simulink model "Sim_Control_Dezvoltare"  (R2022b)
settings: Solver=VariableStepAuto  StartTime=0.0  StopTime=400  RelTol=1e-3
values from neighbouring files (symbols this model uses):
  g = 9.80665    [Date_initializare_SIM.m]
  h = 0.30    (= 0.3)    [Date_initializare_SIM.m]
undefined symbols (not defined in the file or in its folder): X, Y, Z
libraries: sm_lib x175, nesl_utility x70, slpidlib x2
(part 5 of 5)

== matlab function Sim_Control_Dezvoltare/MATLAB Function7 ==
  data: pstar input size=[3,1]; q_bl output size=[1,3]; Tx input; Ty input; Tz input; Rx input; Ry input; Rz input
function q_bl = ikine_rl_f(pstar, Tx, Ty, Tz, Rx, Ry, Rz)
  
    R_DH = rotz(0)*roty(90)*rotx(0);
    T_DH = [0; 0; 0];
    O_DH = [R_DH, T_DH; [0 0 0 1] ];
    
    R_fr = rotz(0)*rotx(0);
    T_fr = [0; 0.047; -0.1805];
    O_fr = [R_fr, T_fr; [0 0 0 1] ];
    
    R_c_corp = rotz(Rx)*roty(Ry)*rotx(Rz);
    T_c_corp = [-Tz; Ty; Tx];
    O_c_corp = [R_c_corp, T_c_corp; [0 0 0 1] ];
        
    B =  O_DH * O_c_corp * O_fr;
    
    pzero = [B(1,4), B(2,4), B(3,4)];
    
    x0_ = pzero(1);
    y0_ = pzero(2);
    z0_ = pzero(3);
    
    x_ = pstar(1);
    y_ = pstar(2);
    z_ = pstar(3);

    Rot = [rotz(Rz)*roty(-Ry)*rotx(-Rx), [0; 0; 0]; [0 0 0 1]];
    Point = [1 0 0 x_-x0_; 0 1 0 y_-y0_; 0 0 1 z_-z0_; 0 0 0 1];
    Origin = [1 0 0 x0_; 0 1 0 y0_; 0 0 1 z0_; 0 0 0 1];
    
    pstar = Origin + Rot*Point;

    x_ = pstar(1,4);
    y_ = pstar(2,4);
    z_ = pstar(3,4);


%     d = sqrt((x_ - x0_)*(x_ - x0_) + (y_ - y0_)*(y_ - y0_) + (z_ - z0_)*(z_ - z0_));
% 
%     th = acos((z_ - z0_)/d) 
%     fis = acos((x_ - x0_)/(d*sin(th)))% + Rz*2*pi/360
% 
%     star = [x0_; y0_; z0_] + rotx(Rx)*roty(-Ry)*rotz(Rz)*(d.*[cos(fis)*sin(th); sin(fis)*sin(th); cos(th)]) 
%     
%     x_ = star(1)
%     y_ = star(2)
%     z_ = star(3)

    
    off = 0.0838;
    L = 0.2;

    m = sqrt((z_ - z0_)*(z_ - z0_));
    n = sqrt( (y_ - y0_)*(y_ - y0_));
    p = sqrt( (y0_ - y_)*(y0_ - y_) + (z0_ - z_)*(z0_ - z_));
    alp0 = atan(n/m);
    alp1 = asin(off/p);
    q1_ = (alp0 - alp1) ;

    x = sqrt((x_ - x0_)*(x_ - x0_));
    r = sqrt(p*p - off*off);
    a = sqrt(r*r + x*x);

    fi = asin((x_ - x0_)/a);

    alpha = acos((a*a + L*L - L*L)/(2*a*L));
    q2_ =  alpha - fi ;
    q3_ = -pi + acos((L*L + L*L - a*a)/(2*L*L)) ;

    q_bl = [q1_, q2_, q3_];

end

== matlab function Sim_Control_Dezvoltare/MATLAB Function18 ==
  data: Fr input; Fl input; centroid output; Rr input; Rl input; pfr input; prl input; prr input; pfl input; rx input; ry input; rz input; rot output
function [centroid, rot]= centroid(Fr, Fl, Rr, Rl, pfr, prl, prr, pfl, rx, ry, rz)

Rot = rotx(rx)*roty(ry)*rotz(rz);
centroid  = (1/(prl + pfl + pfr + prr).*(prl.*Rl + prr.*Rr + pfr.*Fr + pfl.*Fl));
rot = [rx, ry, rz];




end

== matlab function Sim_Control_Dezvoltare/MATLAB Function22 ==
  data: X1 output; A input; B input; t input; d input
function X1 = Traj(A, B, t, d)
  
% t = -1:0.01:1;
% A = [1, 1, 8]';
% B = [1, 10, 8]';


C = 1/2*(A + B);
D = C + [0, 0, d]';

X1 = C + (C - A)*t + (D-C)*(1-t^2);



end

== matlab function Sim_Control_Dezvoltare/MATLAB Function23 ==
  data: X output; A input; B input; t input; d input
function X = Traj(A, B, t, d)
  
% t = -1:0.01:1;
% A = [1, 1, 8]';
% B = [1, 10, 8]';


C = 1/2*(A + B);
D = C + [0, 0, d]';

X = C + (C - A)*t + (D-C)*(1-t^2);



end

== matlab function Sim_Control_Dezvoltare/MATLAB Function24 ==
  data: X output; A input; B input; t input; d input
function X = Traj(A, B, t, d)
  
% t = -1:0.01:1;
% A = [1, 1, 8]';
% B = [1, 10, 8]';


C = 1/2*(A + B);
D = C + [0, 0, d]';

X = C + (C - A)*t + (D-C)*(1-t^2);



end

== matlab function Sim_Control_Dezvoltare/MATLAB Function25 ==
  data: step input; traj output size=[1,2]
function traj = fcn(step)
    
    if step == 0
        step = 1;
    end
    %x = 0:3:1000;
    x = linspace(0,300,100);
    y = 0:0.3:60;
    
    traj = [x(step),0];


end

== matlab function Sim_Control_Dezvoltare/MATLAB Function26 ==
  data: X input; Tx output; Ty output; Tz output; Y input; Z input; R input; Rx output; Ry output; Rz output
function [Tx, Ty, Tz, Rx, Ry, Rz]= Corp(X, Y, Z, R)

Tx = X;
Ty = Y;
Tz = Z;

Rx = R(1,1);
Ry = R(1,2);
Rz = R(1,3);

end

== matlab function Sim_Control_Dezvoltare/MATLAB Function28 ==
  data: X output; A input; B input; t input; d input
function X = Traj(A, B, t, d)
  
% t = -1:0.01:1;
% A = [1, 1, 8]';
% B = [1, 10, 8]';

C = 1/2*(A + B);
D = C + [0, 0, d]';

X = C + (C - A)*t + (D-C)*(1-t^2);



end

== stateflow chart Sim_Control_Dezvoltare/Step Planning Logic3 ==
  settings: updateMethod=DISCRETE  sampleTime=0.1
  state control [function]
    (default) -> (junction 43) : {
        | footRH_prev =  footRH;
        | footLH_prev =  footLH;
        | footRB_prev =  footRB;
        | footLB_prev =  footLB;
        | RH = offRH + [xrefRH;yrefRH;zrefRH];
        |
        | Rot = rotx(rx_out)*roty(ry_out)*rotz(rz_out);
        |
        | footRH = (Rot*RH)
        | }
  state control1 [function]
    (default) -> (junction 139) : {
        | footRH_prev =  footRH;
        | footLH_prev =  footLH;
        | footRB_prev =  footRB;
        | footLB_prev =  footLB;
        |
        | LB = offLB + [xrefLB;yrefLB;zrefLB];
        | Rot = rotx(rx_out)*roty(ry_out)*rotz(rz_out);
        |
        | footLB = (Rot*LB);
        | }
  state control2 [function]
    (default) -> (junction 245) : {
        |
        | footRH_prev =  footRH;
        | footLH_prev =  footLH;
        | footRB_prev =  footRB;
        | footLB_prev =  footLB;
        |
        | LH = offLH + [xrefLH;yrefLH;zrefLH];
        |
        | Rot = rotx(rx_out)*roty(ry_out)*rotz(rz_out);
        | footLH = (Rot*LH);
        |
        | }
  state control3 [function]
    (default) -> (junction 249) : {
        |
        | footRH_prev =  footRH;
        | footLH_prev =  footLH;
        | footRB_prev =  footRB;
        | footLB_prev =  footLB;
        |
        | RB = offRB + [xrefRB;yrefRB;zrefRB];
        | Rot = rotx(rx_out)*roty(ry_out)*rotz(rz_out);
        |
        | footRB = (Rot*RB);
        |
        | }
  state test8
  state Initial
    t = -1;
    timp_traj = t;
    dRH = 0;
    dLB = 0;
    dRB = 0;
    dLH = 0;
    prr = 1;
    prl = 1;
    pfr = 1;
    pfl = 1;
    rx_out = 0.001;
    ry_out = 0.001;
    rz_out = 0.001;
    control;
    control1;
    control2;
    control3;
  state test4
    step = step+1;
  state RightFrontFoot
    xrefRH = stepFwd;
    yrefRH = max(0,stepLat);
    dRH = 0;
    dLB = 0;
    dRB = 0;
    dLH = 0;
    prr = 1;
    prl = 1;
    pfr = 0;
    pfl = 1;
    t = -1;
    rx_out = rx;
    ry_out = ry;
    rz_out = rz;
    timp_traj = t;
    control
  state LeftBackFoot
    xrefLB = stepFwd;
    yrefLB = max(0,stepLat);
    dRH = 0;
    dLB = 0;
    dRB = 0;
    dLH = 0;
    prr = 1;
    prl = 0;
    pfr = 1;
    pfl = 1;
    t = -1;
    timp_traj = t;
    control1
  state timp
    if t<1
    dRH = hs;
    dLB = 0;
    dRB = 0;
    dLH = 0;
    t = t + increment;
    timp_traj = t;
    end
    %if t>=1
    %  if t~=1
    %      t = 1;
    %    timp_traj = t;
    % else
    %   timp_traj = timp_traj + inc
    %end
    %end
  state test
    after(1,sec)
  state test7
    step = step+1;
  state timp1
    if t<1
    dRH = 0;
    dLB = 0;
    dRB = hs;
    dLH = 0;
    t = t + increment;
    timp_traj = t;
    end
  state test1
    after(1,sec)
  state timp2
    if t<1
    dRH = 0;
    dLB = hs;
    dRB = 0;
    dLH = 0;
    t = t + increment;
    timp_traj = t;
    end
  state test6
    step = step+1;
  state test5
    after(1,sec)
  state LeftFrontFoot
    xrefLH = stepFwd;
    yrefLH = max(0,stepLat);
    dRH = 0;
    dLB = 0;
    dRB = 0;
    dLH = 0;
    prr = 1;
    prl = 1;
    pfr = 1;
    pfl = 0;
    t = -1;
    rx_out = rx;
    ry_out = ry;
    rz_out = rz;
    timp_traj = t;
    control2
  state timp3
    if t<1
    dRH = 0;
    dLB = 0;
    dRB = 0;
    dLH = hs;
    t = t + increment;
    timp_traj = t;
    end
  state RightBackFoot
    xrefRB = stepFwd;
    yrefRB= max(0,stepLat);
    dRH = 0;
    dLB = 0;
    dRB = 0;
    dLH = 0;
    prr = 0;
    prl = 1;
    pfr = 1;
    pfl = 1;
    t = -1;
    timp_traj = t;
    control3
  state test2
    after(1,sec)
  (default) -> test8 : % Initialize values
      | {
      | offRH = [0.1805; -0.047-0.0838; -0.3];
      | offLH = [0.1805; 0.047+0.0838; -0.3];
      | offRB = [-0.1805; -0.047-0.0838; -0.3];
      | offLB = [-0.1805; 0.047+0.0838; -0.3];
      | footRH = (offRH);
      | footLH = (offLH);
      | footRB = (offRB);
      | footLB = (offLB);
      | footRH_prev = (offRH);
      | footLH_prev = (offLH);
      | footRB_prev = (offRB);
      | footLB_prev = (offLB);
      |
      | hs = 0.1;
      |
      | tol = 0.01;
      | inc = 0.001;
      | increment = 0.5;
      | t = -1;
      | timp_traj = t;
      | dRH = 0;
      | dLB = 0;
      | dRB = 0;
      | dLH = 0;
      | prr = 1;
      | prl = 1;
      | pfr = 1;
      | pfl = 1;
      | xrefLH = 0; yrefLH = 0; zrefLH = 0;
      | xrefRH = 0; yrefRH = 0; zrefRH = 0;
      | xrefLB = 0; yrefLB = 0; zrefLB = 0;
      | xrefRB = 0; yrefRB = 0; zrefRB = 0;
      | step = 1;
      | rx_out = 0.001;
      | ry_out = 0.001;
      | rz_out = 0.001;
      |
      | control;
      | control1;
      | control2;
      | control3;
      |
      | }
  test8 -> Initial
  Initial -> test4
  test4 -> RightFrontFoot : [err_cg<tol ]
  timp -> timp [order 1] : [ presFR==0]
  test -> timp : [err_cg<tol]
  RightFrontFoot -> test
  timp -> LeftBackFoot [order 2] : [ presFR>0 && t>=1]
  LeftBackFoot -> test1
  test7 -> RightFrontFoot
  timp2 -> timp2 [order 1] : [presRL==0]
  timp1 -> test7 [order 1] : [presRR>0 && t>=1]
  test1 -> timp2 : [err_cg<tol ]
  timp2 -> test6 [order 2] : [ presRL>0 && t>=1]
  test5 -> timp1 : [err_cg<tol ]
  timp1 -> timp1 [order 2] : [presRR==0]
  test6 -> LeftFrontFoot
  RightBackFoot -> test5
  timp3 -> timp3 [order 1] : [presFL==0]
  timp3 -> RightBackFoot [order 2] : [presFL>0 && t>=1]
  test2 -> timp3 : [err_cg<tol]
  LeftFrontFoot -> test2
  data: footRH output size=[3,1]; footLH output size=[3,1]; stepFwd input size=[1,1]; stepLat input size=[1,1]; xRH local; yRH local; zRH local; xLH local; yLH local; zLH local; low local; Kwalk parameter; yrefLH local; zrefLH local; xrefLH local; yrefRH local; zrefRH local; xrefRH local; footRB output size=[3,1]; footLB output size=[3,1]; xLB local; xRB local; xrefLB local; xrefRB local; yLB local; yRB local; yrefLB local; yrefRB local; zLB local; zRB local; zrefLB local; zrefRB local; dRH output size=[1,1]; dLB output size=[1,1]; dRB output size=[1,1]; dLH output size=[1,1]; prr output size=[1,1]; prl output size=[1,1]; pfr output size=[1,1]; pfl output size=[1,1]; footRH_prev output size=[3,1]; footLH_prev output size=[3,1]; footRB_prev output size=[3,1]; footLB_prev output size=[3,1]; offLB local; offLH local; offRB local; offRH local; timp_traj output; t local; hs local double; tol local; presFR input; presFL input; presRR input; presRL input; increment local; err_cg input; step output; R input; rx input; ry input; rz input; rx_out output; ry_out output; rz_out output; RB local; LB local; LB_prev local; LH local; LH_prev local; RB_prev local; RH local; RH_prev local; Rot local; tol_mat local; toll local; inc local

== matlab function Sim_Control_Dezvoltare/MATLAB Function29 ==
  data: Ce_H_RR input; E output; Ce_T_RR input; Ce_C_RR input; Ce_H_RL input; Ce_T_RL input; Ce_C_RL input; Ce_H_FR input; Ce_T_FR input; Ce_C_FR input; Ce_H_FL input; Ce_T_FL input; Ce_C_FL input; Se_H_RR input; Se_T_RR input; Se_C_RR input; Se_H_RL input; Se_T_RL input; Se_C_RL input; Se_H_FR input; Se_T_FR input; Se_C_FR input; Se_H_FL input; Se_T_FL input; Se_C_FL input
function E = fcn(Ce_H_RR, Ce_T_RR, Ce_C_RR, Ce_H_RL, Ce_T_RL, Ce_C_RL, Ce_H_FR, Ce_T_FR, Ce_C_FR, Ce_H_FL, Ce_T_FL, Ce_C_FL, Se_H_RR, Se_T_RR, Se_C_RR, Se_H_RL, Se_T_RL, Se_C_RL, Se_H_FR, Se_T_FR, Se_C_FR, Se_H_FL, Se_T_FL, Se_C_FL)

    Ce = [Ce_H_RR, Ce_T_RR, Ce_C_RR, Ce_H_RL, Ce_T_RL, Ce_C_RL, Ce_H_FR, Ce_T_FR, Ce_C_FR, Ce_H_FL, Ce_T_FL, Ce_C_FL]';
    Se = [Se_H_RR, Se_T_RR, Se_C_RR, Se_H_RL, Se_T_RL, Se_C_RL, Se_H_FR, Se_T_FR, Se_C_FR, Se_H_FL, Se_T_FL, Se_C_FL]';

    E_vect = Ce - Se;

    E = sum(E_vect);


end
